simulink model "DKM"  (R2015a)
settings: Solver=ode5  StartTime=0.0  StopTime=10.0  FixedStep=0.01  RelTol=1e-3
values from neighbouring files (symbols this model uses):
  a = 0.15    [Init.m]    (also in lyapu.m; plotKinematic.m = 0.13)
  beta0 = (K-1)*0.05    [plotKinematic.m]
  beta_dot = 0    [plotKinematic.m]
  phi_dot = 5    [plotKinematic.m]
  r = 0.1    [Init.m]    (also in plotKinematic.m)
settings Model: Creator=tgvo  LastModifiedBy=tgvo

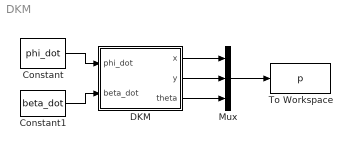
== system DKM ==
  Constant : Constant  Value=phi_dot
  Constant1 : Constant  Value=beta_dot
  DKM : Subsystem  mask{beta0=beta0, a=a, r=r}
      mask prompts: beta0 "Initial value of Beta"
  Mux : Mux  Inputs=3
  To Workspace : ToWorkspace  VariableName=p  SampleTime=-1
  wires:
  Constant/1 -> DKM/1(phi_dot)
  Constant1/1 -> DKM/2(beta_dot)
  DKM/3(theta) -> Mux/3
  DKM/2(y) -> Mux/2
  DKM/1(x) -> Mux/1
  Mux/1 -> To Workspace/1

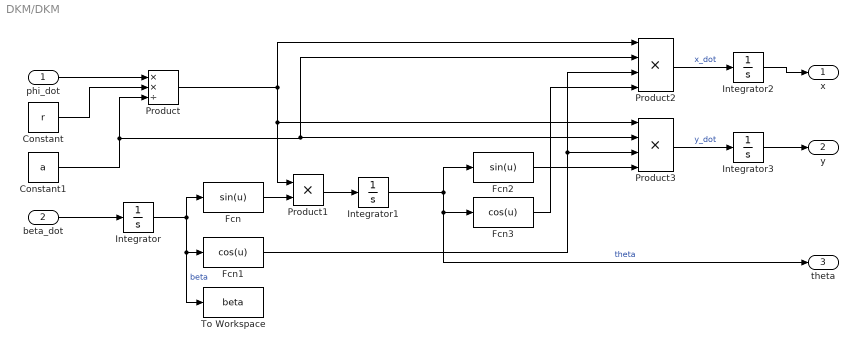
== system DKM/DKM ==
  phi_dot : Inport
  beta_dot : Inport  Port=2
  Constant : Constant  Value=r
  Constant1 : Constant  Value=a
  Fcn : Fcn  Expr=sin(u)
  Fcn1 : Fcn  Expr=cos(u)
  Fcn2 : Fcn  Expr=sin(u)
  Fcn3 : Fcn  Expr=cos(u)
  Integrator : Integrator  InitialCondition=beta0
  Integrator1 : Integrator
  Integrator2 : Integrator
  Integrator3 : Integrator
  Product : Product  Inputs=**/
  Product1 : Product
  Product2 : Product  Inputs=4
  Product3 : Product  Inputs=4
  To Workspace : ToWorkspace  VariableName=beta  SampleTime=-1
  x : Outport
  y : Outport  Port=2
  theta : Outport  Port=3
  wires:
  Constant/1 -> Product/2
  phi_dot/1 -> Product/1
  beta_dot/1 -> Integrator/1
  Integrator/1 -> Fcn/1, To Workspace/1, Fcn1/1  "beta"
  Fcn/1 -> Product1/2
  Product/1 -> Product3/1, Product1/1, Product2/1
  Product1/1 -> Integrator1/1
  Integrator1/1 -> Fcn2/1, theta/1, Fcn3/1  "theta"
  Constant1/1 -> Product3/2, Product2/2, Product/3
  Fcn1/1 -> Product3/3, Product2/3
  Fcn3/1 -> Product2/4
  Fcn2/1 -> Product3/4
  Product2/1 -> Integrator2/1  "x_dot"
  Product3/1 -> Integrator3/1  "y_dot"
  Integrator3/1 -> y/1
  Integrator2/1 -> x/1
